simulink model "boost_sim2"  (R2025b)
settings: Solver=VariableStepAuto  StartTime=0.0  StopTime=0.01  FixedStep=Tstep  RelTol=1e-3
values from neighbouring files (symbols this model uses):
  Duty = (1-invDuty_setp)*100    (= 18.5)    [boost_converter_main.m]
  PWMenable = 1    [boost_converter_main.m]
  R_Vin = 30*10^-3    (= 0.03)    [boost_converter_main.m]
  Rload = 400    [boost_converter_main.m]
  Tsw = 1/Fsw    (= 2e-05)    [boost_converter_main.m]
libraries: fl_lib x10, ee_lib x9, nesl_utility x9, simulink x1
settings Model: Creator=jobme  LastModifiedBy=Job
settings SolverCC: DaesscMode=Balanced
settings HardwareCC: ProdHWDeviceType=AMD->x86-64 (Windows64)
settings SFSimCC: UsePrecompiledLibraries=Avoid  SimTargetLang=C++  GPUAcceleration=on  SimDLTargetLibrary=cudnn

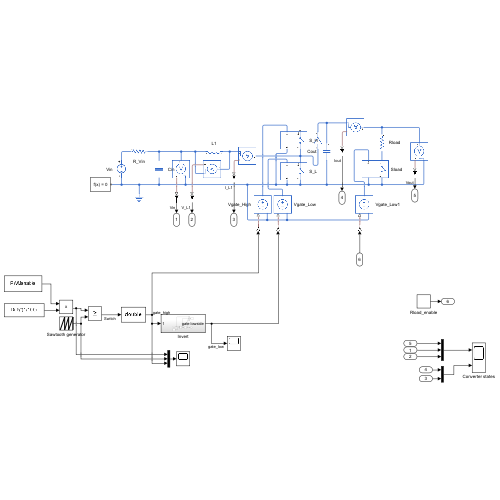
[thumbnail: Simulink's stored preview of the top-level diagram]
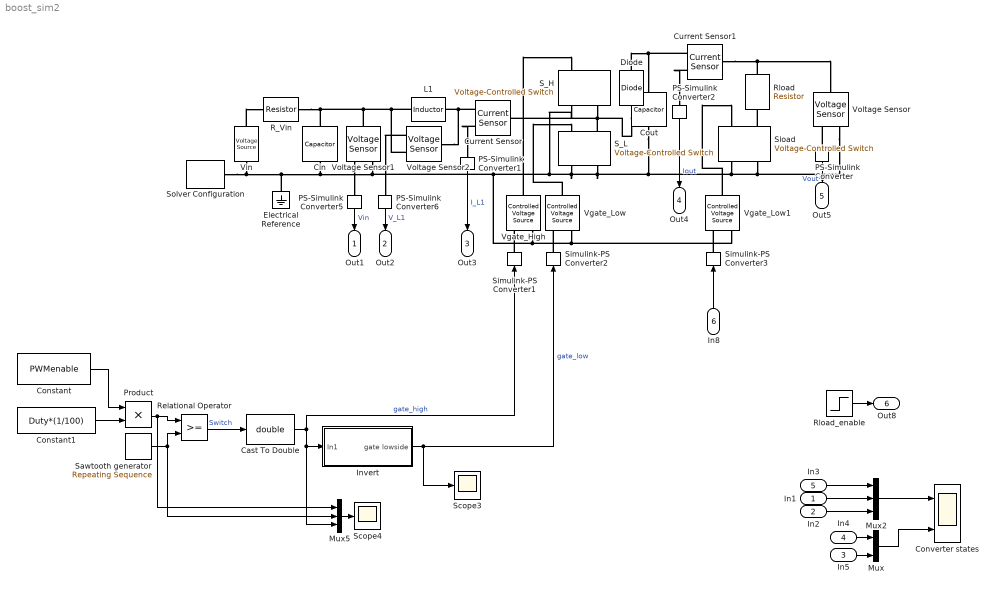
== system boost_sim2 ==
  In1 : Inport
  In2 : Inport  Port=2
  In5 : Inport  Port=3
  In4 : Inport  Port=4
  In3 : Inport  Port=5
  In8 : Inport  Port=6
  Cast To Double : DataTypeConversion  OutDataTypeStr=double  SaturateOnIntegerOverflow=off  RndMeth=Floor
  Cin : ee_lib/Passive/Capacitor  cap_option=ee.enum.passive.capacitor.capOption.const  c=Cin F  Cvec=[1e-05, 1e-06] F  Vvec=[0, 10] V  CV_table_symmetry=ee.enum.passive.capacitor.tableSymmetry.yes  f_vec=[1, 10] kHz  DFext_vec=[.8, 1.2]  enable_C_tol=ee.enum.toleranceApplication.none  averaging_period=0 s  C_tol=5  tol_distribution=ee.enum.toleranceDistribution.uniform  nSigma=4  r=0 Ohm  g=0 1/Ohm  enable_operating_limits=ee.enum.enable.no  operating_limit_action=ee.enum.passive.reportOpLim.warn  max_working_voltage_range=[-25, 25] V  power_rating=1 W  maxTemperature=85 degC  thermalEnable=false  thermalMass=1 J/K  i_specify=off  i_priority=None  i=0 A  i_nominal_specify=off  i_nominal_value=1  i_nominal_unit=A  v_specify=off  v_priority=None  v=Vinit_Cin V  v_nominal_specify=off  v_nominal_value=1  v_nominal_unit=V  vc_specify=off  vc_priority=High  vc=Vinit_Cin V  vc_nominal_specify=off  vc_nominal_value=1  vc_nominal_unit=V  T_specify=off  T_priority=None  T=298.15 K  T_nominal_specify=off  T_nominal_value=1  T_nominal_unit=K
  Constant : Constant  Value=PWMenable
  Constant1 : Constant  Value=Duty*(1/100)
  Converter states : Scope  NumInputPorts=2
      settings: ActiveDisplayYMinimum=-1  ActiveDisplayYMaximum=1  DataLoggingDecimation=32  DataLoggingVariableName=states
  Cout : ee_lib/Passive/Capacitor  cap_option=ee.enum.passive.capacitor.capOption.const  c=Cout F  Cvec=[1e-05, 1e-06] F  Vvec=[0, 10] V  CV_table_symmetry=ee.enum.passive.capacitor.tableSymmetry.yes  f_vec=[1, 10] kHz  DFext_vec=[.8, 1.2]  enable_C_tol=ee.enum.toleranceApplication.none  averaging_period=0 s  C_tol=5  tol_distribution=ee.enum.toleranceDistribution.uniform  nSigma=4  r=0 Ohm  g=0 1/Ohm  enable_operating_limits=ee.enum.enable.no  operating_limit_action=ee.enum.passive.reportOpLim.warn  max_working_voltage_range=[-25, 25] V  power_rating=1 W  maxTemperature=85 degC  thermalEnable=false  thermalMass=1 J/K  i_specify=off  i_priority=None  i=0 A  i_nominal_specify=off  i_nominal_value=1  i_nominal_unit=A  v_specify=off  v_priority=None  v=Vinit_Cout V  v_nominal_specify=off  v_nominal_value=1  v_nominal_unit=V  vc_specify=off  vc_priority=High  vc=Vinit_Cout V  vc_nominal_specify=off  vc_nominal_value=1  vc_nominal_unit=V  T_specify=off  T_priority=None  T=298.15 K  T_nominal_specify=off  T_nominal_value=1  T_nominal_unit=K
  Current Sensor : fl_lib/Electrical/Electrical Sensors/Current Sensor
  Current Sensor1 : fl_lib/Electrical/Electrical Sensors/Current Sensor
  Diode : fl_lib/Electrical/Electrical Elements/Diode  Vf=0.6 V  Ron=0.3 Ohm  Goff=1e-8 1/Ohm  i_specify=off  i_priority=None  i=0 A  i_nominal_specify=off  i_nominal_value=1  i_nominal_unit=A  v_specify=off  v_priority=None  v=0 V  v_nominal_specify=off  v_nominal_value=1  v_nominal_unit=V
  Electrical Reference : fl_lib/Electrical/Electrical Elements/Electrical Reference
  Invert : Subsystem
  L1 : ee_lib/Passive/Inductor  l=L1 H  enable_L_tol=ee.enum.toleranceApplication.none  L_tol=20  tol_distribution=ee.enum.toleranceDistribution.uniform  nSigma=4  r=R_L1 Ohm  g=1e-9 1/Ohm  enable_operating_limits=ee.enum.enable.no  operating_limit_action=ee.enum.passive.reportOpLim.warn  max_working_current=1 A  power_rating=1 W  i_L_specify=off  i_L_priority=High  i_L=Iinit_L1 A  i_L_nominal_specify=off  i_L_nominal_value=1  i_L_nominal_unit=A
  Mux : Mux  Inputs=2
  Mux2 : Mux  Inputs=3
  Mux5 : Mux  Inputs=3
  PS-Simulink Converter{,1..2,5..6} (5 alike) : nesl_utility/PS-Simulink Converter  PhysicalDomain=network_engine_domain  SubClassName=ps_output  LeftPortType=input  RightPortType=output  PseudoPeriodic=off  Frequencies=[]  VectorFormat=inherit  Unit=inherit  AffineConversion=off
  Product : Product
  R_Vin : ee_lib/Passive/Resistor  R=R_Vin Ohm  enable_R_tol=0  R_tol=0.1  tol_distribution=1  nSigma=4  enable_operating_limits=0  operating_limit_action=2  power_rating=1 W  max_working_voltage=100 V  noise_mode=0  Tdevice=25 degC  sample_time=1e-3 s  repeatability=1  user_seed=0  auto_seed=3241354618  power_derating_T1=70 degC  power_derating_T2=155 degC  operating_temperature_range_vec=[-50, 150] degC  alpha=3.93e-3 1/K  Tmeas=25 degC  thermal_mass=100 J/K  temperature_specify=off  temperature_priority=High  temperature=298.15 K  temperature_nominal_specify=off  temperature_nominal_value=1  temperature_nominal_unit=K
  Relational Operator : RelationalOperator  OutDataTypeStr=boolean  RndMeth=Simplest  InputSameDT=off
  Rload : ee_lib/Passive/Resistor  R=Rload Ohm  enable_R_tol=ee.enum.toleranceApplication.none  R_tol=5  tol_distribution=ee.enum.toleranceDistribution.uniform  nSigma=4  enable_operating_limits=ee.enum.enable.no  operating_limit_action=ee.enum.passive.reportOpLim.warn  power_rating=1 W  max_working_voltage=100 V  noise_mode=ee.enum.sources.noise.Disabled  Tdevice=25 degC  sample_time=1e-3 s  repeatability=ee.enum.ic.repeatability.notRepeatable  user_seed=0  auto_seed=3499211588  power_derating_T1=70 degC  power_derating_T2=155 degC  operating_temperature_range_vec=[-50, 150] degC  alpha=3.93e-3 1/K  Tmeas=25 degC  thermal_mass=100 J/K  temperature_specify=off  temperature_priority=High  temperature=298.15 K  temperature_nominal_specify=off  temperature_nominal_value=1  temperature_nominal_unit=K
  Rload_enable : Step  Time=0  SampleTime=0
  S_H : ee_lib/Additional Components/SPICE Passives/Voltage-Controlled Switch  SWITCH_model=ee.enum.switches.switchModelVoltage.resistance  VON=1 V  VOFF=0 V  VT=1 V  VH=0 V  RON=0.0001 Ohm  ROFF_res=1e6 Ohm  Roff_gmin=ee.enum.switches.offResistance.no  ROFF=10e6 Ohm  TD=0 s
      settings: InternalSimscapePortConfiguration="{\"Bottom\":[],\"Left\":[{\"id\":\"p1\",\"label\":\"1+\",\"type\":\"foundation.electrical.electrical\"},{\"id\":\"p2\",\"label\":\"2+\",\"type\":\"foundation.electrical.electrical\"}],\"Right\":[{\"id\":\"n1\",\"label\":\"1-\",\"type\":\"foundation.electrical.electrical\"},{\"id\":\"n2\",\"label\":\"2-\",\"type\":\"foundation.electrical.electrical\"}],\"Top\":[]}"
  S_L : ee_lib/Additional Components/SPICE Passives/Voltage-Controlled Switch  SWITCH_model=ee.enum.switches.switchModelVoltage.resistance  VON=1 V  VOFF=0 V  VT=1 V  VH=0 V  RON=0.0001 Ohm  ROFF_res=1e6 Ohm  Roff_gmin=ee.enum.switches.offResistance.no  ROFF=10e6 Ohm  TD=0 s
      settings: InternalSimscapePortConfiguration="{\"Bottom\":[],\"Left\":[{\"id\":\"p1\",\"label\":\"1+\",\"type\":\"foundation.electrical.electrical\"},{\"id\":\"p2\",\"label\":\"2+\",\"type\":\"foundation.electrical.electrical\"}],\"Right\":[{\"id\":\"n1\",\"label\":\"1-\",\"type\":\"foundation.electrical.electrical\"},{\"id\":\"n2\",\"label\":\"2-\",\"type\":\"foundation.electrical.electrical\"}],\"Top\":[]}"
  Sawtooth generator : simulink/Sources/Repeating Sequence  rep_seq_t=[0 Tsw]  rep_seq_y=[0 1]
  Scope3 : Scope
      settings: ActiveDisplayYMinimum=-0.12499999999999997  ActiveDisplayYMaximum=1.125  DataLoggingVariableName=ScopeData4
  Scope4 : Scope
      settings: ActiveDisplayYMinimum=-0.12499999999999997  ActiveDisplayYMaximum=1.125  DataLoggingVariableName=ScopeData5
  Simulink-PS Converter1 : nesl_utility/Simulink-PS Converter  PhysicalDomain=network_engine_domain  SubClassName=ps_input  LeftPortType=input  RightPortType=output  PseudoPeriodic=off  Frequencies=[]  NoiseDistribution=none  NoiseParameters=[]  Unit=1  AffineConversion=off  FilteringAndDerivatives=provide  SimscapeFilterOrder=1  InputFilterTimeConstant=0.001  UdotUserProvided=0
  Simulink-PS Converter2 : nesl_utility/Simulink-PS Converter  PhysicalDomain=network_engine_domain  SubClassName=ps_input  LeftPortType=input  RightPortType=output  PseudoPeriodic=off  Frequencies=[]  NoiseDistribution=none  NoiseParameters=[]  Unit=1  AffineConversion=off  FilteringAndDerivatives=provide  SimscapeFilterOrder=1  InputFilterTimeConstant=0.001  UdotUserProvided=0
  Simulink-PS Converter3 : nesl_utility/Simulink-PS Converter  PhysicalDomain=network_engine_domain  SubClassName=ps_input  LeftPortType=input  RightPortType=output  PseudoPeriodic=off  Frequencies=[]  NoiseDistribution=none  NoiseParameters=[]  Unit=1  AffineConversion=off  FilteringAndDerivatives=provide  SimscapeFilterOrder=1  InputFilterTimeConstant=0.001  UdotUserProvided=0
  Sload : ee_lib/Additional Components/SPICE Passives/Voltage-Controlled Switch  SWITCH_model=ee.enum.switches.switchModelVoltage.transition  VON=1 V  VOFF=0 V  VT=1 V  VH=0 V  RON=0.0001 Ohm  ROFF_res=1e6 Ohm  Roff_gmin=ee.enum.switches.offResistance.no  ROFF=10e6 Ohm  TD=0 s
      settings: InternalSimscapePortConfiguration="{\"Bottom\":[],\"Left\":[{\"id\":\"p1\",\"label\":\"1+\",\"type\":\"foundation.electrical.electrical\"},{\"id\":\"p2\",\"label\":\"2+\",\"type\":\"foundation.electrical.electrical\"}],\"Right\":[{\"id\":\"n1\",\"label\":\"1-\",\"type\":\"foundation.electrical.electrical\"},{\"id\":\"n2\",\"label\":\"2-\",\"type\":\"foundation.electrical.electrical\"}],\"Top\":[]}"
  Solver Configuration : nesl_utility/Solver Configuration  PhysicalDomain=network_engine_domain  SubClassName=solver  LeftPortType=input  RightPortType=generic  Tones=[]  Harmonics=[]  SimulateNoise=off  Profile=off  UseLocalSampling=off  EnableSwitchedLinearOptims=on  FrequencyDomain=off  UseCCode=off  RelTol=0.001  AbsTol=0.001  MinStep=1e-09  ToWorkspace=off  RevertToSquareIcSolve=off  NumHomotopyIterations=100  PhasorMode=off  PhasorModeNumHarmonics=1  ConsistencySolver=NEWTON_XTOL_AFTER_FTOL  IndexReductionMethod=DerivativeReplacement  DoDC=off  ResidualTolerance=1e-09  ConsistencyTolSource=GLOBAL  ConsistencyAbsTol=0.001  ConsistencyRelTol=0.001  ConsistencyTolFactor=0.001  UseLocalSolver=off  LocalSolverChoice=NE_BACKWARD_EULER_ADVANCER  ResolveIndetEquations=off  FunctionEvalNumThread=1  LocalSolverSampleTime=Tstep  DoFixedCost=off  MaxNonlinIter=3  MaxModeIter=2  ComputeImpulses=off  ImpulseIterations=2  LinearAlgebra=auto  LinearAlgebraNumThread=0  EquationFormulation=NE_TIME_EF  DelaysMemoryBudget=1024  AutomaticFiltering=off  FilteringTimeConstant=0.001  PartitionStorageMethod=AS_NEEDED  PartitionMemoryBudget=1024  PartitionMethod=ROBUST  MultibodyUseLocalSolver=off  MultibodyLocalSolverChoice=ODE1  MultibodyLocalSolverSampleTime=0.001
  Vgate_High : fl_lib/Electrical/Electrical Sources/Controlled Voltage Source
  Vgate_Low : fl_lib/Electrical/Electrical Sources/Controlled Voltage Source
  Vgate_Low1 : fl_lib/Electrical/Electrical Sources/Controlled Voltage Source
  Vin : ee_lib/Sources/Voltage Source  dc_voltage=Vin V  ac_voltage=0 V  ac_shift=0 rad  ac_frequency=0 Hz  noise_mode=0  PSD=0 V^2/Hz  sample_time=1e-3 s  repeatability=1  user_seed=0  auto_seed=3046698749  i_specify=off  i_priority=None  i=0 A  i_nominal_specify=off  i_nominal_value=1  i_nominal_unit=A  v_specify=off  v_priority=None  v=0 V  v_nominal_specify=off  v_nominal_value=1  v_nominal_unit=V
  Voltage Sensor : fl_lib/Electrical/Electrical Sensors/Voltage Sensor
  Voltage Sensor1 : fl_lib/Electrical/Electrical Sensors/Voltage Sensor
  Voltage Sensor2 : fl_lib/Electrical/Electrical Sensors/Voltage Sensor
  Out1 : Outport
  Out2 : Outport  Port=2
  Out3 : Outport  Port=3
  Out4 : Outport  Port=4
  Out5 : Outport  Port=5
  Out8 : Outport  Port=6
  wires:
  Mux/1 -> Converter states/2
  Mux2/1 -> Converter states/1
  PS-Simulink Converter5/1 -> Out1/1  "Vin"
  In1/1 -> Mux2/2
  PS-Simulink Converter6/1 -> Out2/1  "V_L1"
  In2/1 -> Mux2/3
  PS-Simulink Converter/1 -> Out5/1  "Vout"
  PS-Simulink Converter2/1 -> Out4/1  "Iout"
  In3/1 -> Mux2/1
  In4/1 -> Mux/1
  PS-Simulink Converter1/1 -> Out3/1  "I_L1"
  In5/1 -> Mux/2
  In8/1 -> Simulink-PS Converter3/1
  Relational Operator/1 -> Cast To Double/1  "Switch"
  Sawtooth generator/1 -> Mux5/2, Relational Operator/2
  Product/1 -> Mux5/1, Relational Operator/1
  Constant/1 -> Product/1
  Rload_enable/1 -> Out8/1
  Cast To Double/1 -> Simulink-PS Converter1/1, Mux5/3, Invert/1(In1)  "gate_high"
  Invert/1(gate lowside) -> Simulink-PS Converter2/1, Scope3/1  "gate_low"
  Constant1/1 -> Product/2
  Mux5/1 -> Scope4/1
  connections:
  Cin/LConn1 -- R_Vin/RConn1 -- Voltage Sensor2/RConn2 -- L1/RConn1 -- Voltage Sensor1/LConn1
  Vin/RConn1 -- Solver Configuration/RConn1 -- Electrical Reference/LConn1 -- Vgate_Low1/RConn2 -- Vgate_Low/RConn2 -- Vgate_High/RConn2 -- S_H/RConn1 -- S_L/RConn1 -- S_L/RConn2 -- Sload/RConn1 -- Sload/RConn2 -- Voltage Sensor/RConn2 -- Cout/RConn1 -- Voltage Sensor1/RConn2 -- Cin/RConn1
  Rload/LConn1 -- Voltage Sensor/LConn1 -- Current Sensor1/LConn1
  PS-Simulink Converter/LConn1 -- Voltage Sensor/RConn1
  Voltage Sensor2/LConn1 -- Current Sensor/RConn2 -- L1/LConn1
  Current Sensor1/RConn1 -- PS-Simulink Converter2/LConn1
  Current Sensor1/RConn2 -- Diode/RConn1 -- Cout/LConn1
  Voltage Sensor1/RConn1 -- PS-Simulink Converter5/LConn1
  Voltage Sensor2/RConn1 -- PS-Simulink Converter6/LConn1
  Current Sensor/RConn1 -- PS-Simulink Converter1/LConn1
  Vin/LConn1 -- R_Vin/LConn1
  S_L/LConn2 -- Diode/LConn1 -- S_H/RConn2 -- Current Sensor/LConn1
  Vgate_High/LConn1 -- S_H/LConn1
  Vgate_Low/LConn1 -- S_L/LConn1
  Simulink-PS Converter1/RConn1 -- Vgate_High/RConn1
  Simulink-PS Converter2/RConn1 -- Vgate_Low/RConn1
  Sload/LConn2 -- Rload/RConn1
  Vgate_Low1/LConn1 -- Sload/LConn1
  Simulink-PS Converter3/RConn1 -- Vgate_Low1/RConn1

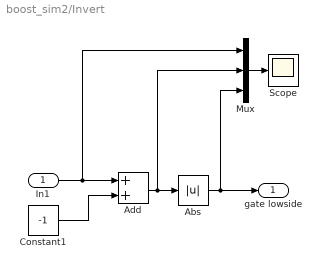
== system boost_sim2/Invert ==
  In1 : Inport
  Abs : Abs  SaturateOnIntegerOverflow=off
  Add : Sum
  Constant1 : Constant  Value=-1
  Mux : Mux  Inputs=3
  Scope : Scope
      settings: DataLoggingVariableName=ScopeData2
  gate lowside : Outport
  wires:
  Constant1/1 -> Add/2
  Add/1 -> Mux/2, Abs/1
  In1/1 -> Mux/1, Add/1
  Abs/1 -> Mux/3, gate lowside/1
  Mux/1 -> Scope/1
